simulink model "closedLoop"  (R2021b)
settings: Solver=VariableStepAuto  StartTime=0.0  StopTime=10.0  RelTol=1e-3
libraries: simulink x1
settings Model: Creator=Asus  LastModifiedBy=Asus

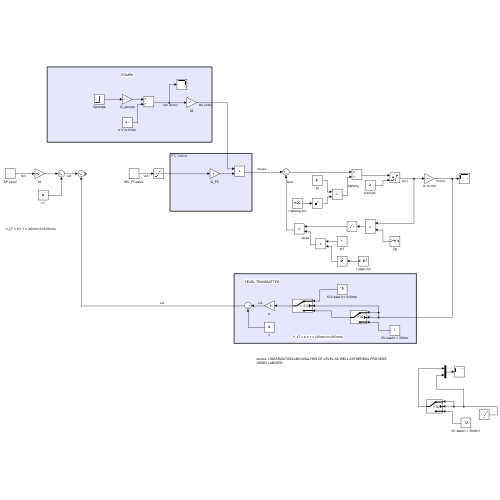
[thumbnail: Simulink's stored preview of the top-level diagram]
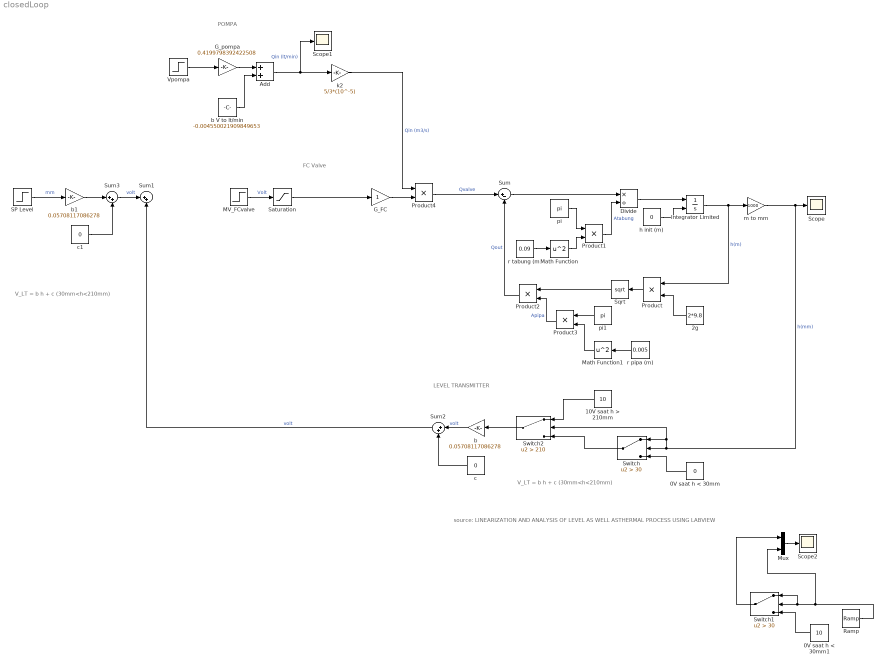
== system closedLoop ==
  note: V_LT = b h + c (30mm<h<210mm)
  note: LEVEL TRANSMITTER
  note: FC Valve
  note: POMPA
  note: source: LINEARIZATION AND ANALYSIS OF LEVEL AS WELL ASTHERMAL PROCESS USING LABVIEW
  note: V_LT = b h + c (30mm<h<210mm)
  0V saat h < 30mm : Constant  Value=0
  0V saat h < 30mm1 : Constant  Value=10
  10V saat h > 210mm : Constant  Value=10
  2g : Constant  Value=2*9.8
  Add : Sum
  Divide : Product  Inputs=*/
  G_FC : Gain
  G_pompa : Gain  Gain=0.4199798392422508
  Integrator Limited : Integrator  InitialConditionSource=external  LimitOutput=on  UpperSaturationLimit=1  LowerSaturationLimit=0
  MV_FCvalve : Step  SampleTime=0
  Math Function : Math  Operator=square  SaturateOnIntegerOverflow=on
  Math Function1 : Math  Operator=square  SaturateOnIntegerOverflow=on
  Mux : Mux  Inputs=2
  Product{,1..4} (5 alike) : Product
  Ramp : simulink/Sources/Ramp  slope=10  start=0  InitialOutput=0
  SP Level : Step  SampleTime=0
  Saturation : Saturate  UpperLimit=10  LowerLimit=0
  Scope : Scope
  Scope1 : Scope
  Scope2 : Scope
  Sqrt : Sqrt  SaturateOnIntegerOverflow=on
  Sum : Sum  Inputs=|+-
  Sum1 : Sum  Inputs=|++
  Sum2 : Sum  Inputs=|++
  Sum3 : Sum  Inputs=|++
  Switch : Switch  Criteria=u2 > Threshold  Threshold=30
  Switch1 : Switch  Criteria=u2 > Threshold  Threshold=30
  Switch2 : Switch  Criteria=u2 > Threshold  Threshold=210
  Vpompa : Step  After=10  SampleTime=0
  b : Gain  Gain=0.05708117086278
  b V to lt/min : Constant  Value=-0.004550021909849653
  b1 : Gain  Gain=0.05708117086278
  c : Constant  Value=0
  c1 : Constant  Value=0
  h init (m) : Constant  Value=0
  k2 : Gain  Gain=5/3*(10^-5)
  m to mm : Gain  Gain=1000
  pi : Constant  Value=pi
  pi1 : Constant  Value=pi
  r pipa (m) : Constant  Value=0.005
  r tabung (m) : Constant  Value=0.09
  wires:
  Sum/1 -> Divide/1
  Divide/1 -> Integrator Limited/1
  Product/1 -> Sqrt/1
  2g/1 -> Product/2
  Sqrt/1 -> Product2/1
  Product2/1 -> Sum/2  "Qout"
  h init (m)/1 -> Integrator Limited/2
  Product1/1 -> Divide/2  "Atabung"
  pi/1 -> Product1/1
  Math Function/1 -> Product1/2
  r tabung (m)/1 -> Math Function/1
  r pipa (m)/1 -> Math Function1/1
  Product3/1 -> Product2/2  "Apipa"
  pi1/1 -> Product3/1
  Math Function1/1 -> Product3/2
  G_pompa/1 -> Add/1
  Add/1 -> Scope1/1, k2/1  "Qin (lt/min)"
  b V to lt/min/1 -> Add/2
  k2/1 -> Product4/1  "Qin (m3/s)"
  Product4/1 -> Sum/1  "Qvalve"
  MV_FCvalve/1 -> Saturation/1  "Volt"
  G_FC/1 -> Product4/2
  SP Level/1 -> b1/1  "mm"
  b1/1 -> Sum3/1
  Sum2/1 -> Sum1/2  "volt"
  Integrator Limited/1 -> Product/1, m to mm/1  "h(m)"
  m to mm/1 -> Switch2/2, Switch/1, Switch/2, Scope/1  "h(mm)"
  Vpompa/1 -> G_pompa/1
  Saturation/1 -> G_FC/1
  0V saat h < 30mm/1 -> Switch/3
  0V saat h < 30mm1/1 -> Switch1/3
  Ramp/1 -> Mux/2, Switch1/1, Switch1/2
  Mux/1 -> Scope2/1
  Switch1/1 -> Mux/1
  Switch/1 -> Switch2/3
  10V saat h > 210mm/1 -> Switch2/1
  Switch2/1 -> b/1
  b/1 -> Sum2/1  "volt"
  c/1 -> Sum2/2
  c1/1 -> Sum3/2
  Sum3/1 -> Sum1/1  "volt"
